simulink model "psd_db"  (R2020a)
settings: Solver=FixedStepDiscrete  StartTime=0.0  StopTime=inf  RelTol=1e-3
InitFcn:
  | spectrum_fft_setup;
  | load('data.mat');
libraries: simulink x3, hdlsllib x1
settings Model: DataTypeOverride=Off  Creator=rgb11127  LastModifiedBy=david
settings DataIOCC: SaveOutput=off  SaveTime=off  ReturnWorkspaceOutputs=off
settings OptimizationCC: BlockReduction=off  ConditionallyExecuteInputs=off  DefaultParameterBehavior=Inlined
settings DebuggingCC: AlgebraicLoopMsg=error  SingleTaskRateTransMsg=error  PregeneratedLibrarySubsystemCodeDiagnostic=none  ArithmeticOperatorsInVariantConditions=warning
settings HardwareCC: ProdBitPerPointer=32  ProdBitPerSizeT=32  ProdBitPerPtrDiffT=32  ProdLargestAtomicFloat=None  ProdIntDivRoundTo=Undefined  ProdEndianess=Unspecified  ProdWordSize=32  ProdHWDeviceType=ASIC/FPGA->ASIC/FPGA  TargetBitPerPointer=64  TargetBitPerSizeT=64  TargetBitPerPtrDiffT=64  TargetLongLongMode=on  TargetIntDivRoundTo=Zero  TargetEndianess=LittleEndian  TargetWordSize=64  TargetHWDeviceType=Custom Processor->MATLAB Host Computer  ProdEqTarget=off
settings SFSimCC: SimUseLocalCustomCode=off  CustomCodeUndefinedFunction=UseInterfaceOnly
settings RTWCC: RTWUseLocalCustomCode=off

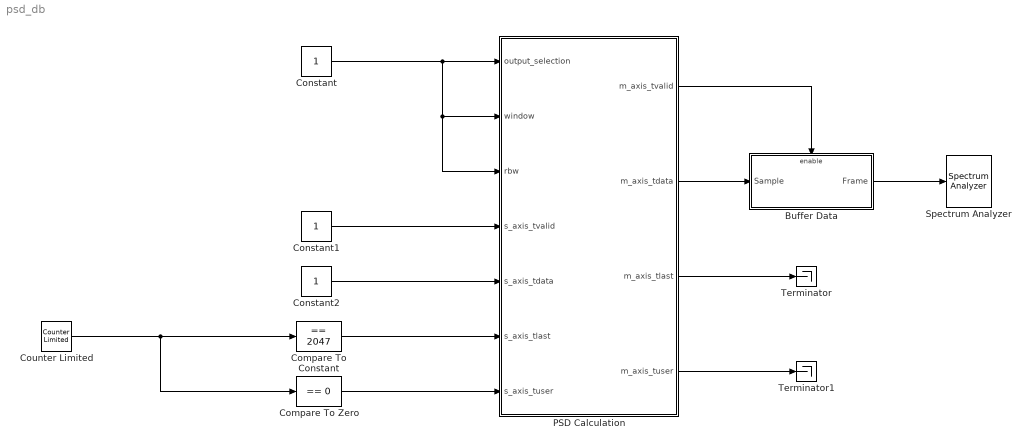
== system psd_db ==
  Buffer Data : Subsystem
  Compare To Constant : simulink/Logic and Bit Operations/Compare To Constant  relop===  const=2047  OutDataTypeStr=boolean
  Compare To Zero : simulink/Logic and Bit Operations/Compare To Zero  relop===  OutDataTypeStr=boolean
  Constant : Constant  OutDataTypeStr=uint32  SampleTime=1/256e6
  Constant1 : Constant  OutDataTypeStr=boolean  SampleTime=-1
  Constant2 : Constant  OutDataTypeStr=uint32  SampleTime=-1
  Counter Limited : simulink/Sources/Counter Limited  uplimit=2047  tsamp=-1
  PSD Calculation : Subsystem  TreatAsAtomicUnit=on
  Spectrum Analyzer : SpectrumAnalyzer  IsFrequencyInputMode=1
  Terminator : Terminator
  Terminator1 : Terminator
  wires:
  Constant/1 -> PSD Calculation/3(rbw), PSD Calculation/2(window), PSD Calculation/1(output_selection)
  PSD Calculation/2(m_axis_tdata) -> Buffer Data/1(Sample)
  PSD Calculation/1(m_axis_tvalid) -> Buffer Data/Enable
  PSD Calculation/3(m_axis_tlast) -> Terminator/1
  PSD Calculation/4(m_axis_tuser) -> Terminator1/1
  Counter Limited/1 -> Compare To Constant/1, Compare To Zero/1
  Compare To Constant/1 -> PSD Calculation/6(s_axis_tlast)
  Constant1/1 -> PSD Calculation/4(s_axis_tvalid)
  Buffer Data/1(Frame) -> Spectrum Analyzer/1
  Compare To Zero/1 -> PSD Calculation/7(s_axis_tuser)
  Constant2/1 -> PSD Calculation/5(s_axis_tdata)

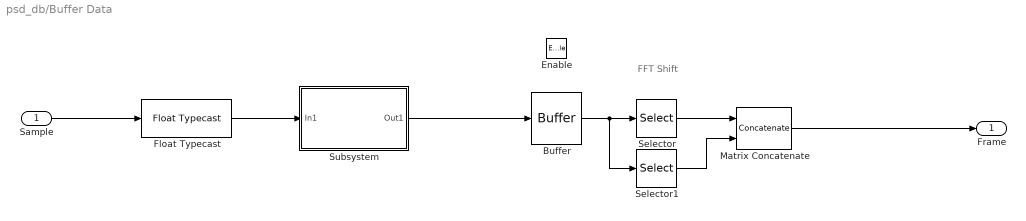
== system psd_db/Buffer Data ==
  note: FFT Shift
  Sample : Inport
  Enable : EnablePort
  Buffer : Buffer  N=2^11  OutputFrames=off
  Float Typecast : FloatTypecast
  Matrix Concatenate : Concatenate  Mode=Multidimensional array
  Selector : Selector  NumberOfDimensions=2  InputPortWidth=3  IndexOptions=Index vector (dialog),Index vector (dialog)  Indices=[1025:1:2048],1  OutputSizes=1,1
  Selector1 : Selector  NumberOfDimensions=2  InputPortWidth=3  IndexOptions=Index vector (dialog),Index vector (dialog)  Indices=[1:1:1024],1  OutputSizes=1,1
  Subsystem : Subsystem  Variant=on  VariantControlMode=Label  VariantControl=Variant1  LabelModeActiveChoice=Variant1
  Frame : Outport  VectorParamsAs1DForOutWhenUnconnected=off
  wires:
  Subsystem/1(" Out1") -> Buffer/1
  Sample/1 -> Float Typecast/1
  Selector1/1 -> Matrix Concatenate/2
  Matrix Concatenate/1 -> Frame/1
  Selector/1 -> Matrix Concatenate/1
  Buffer/1 -> Selector1/1, Selector/1
  Float Typecast/1 -> Subsystem/1("In1 ")

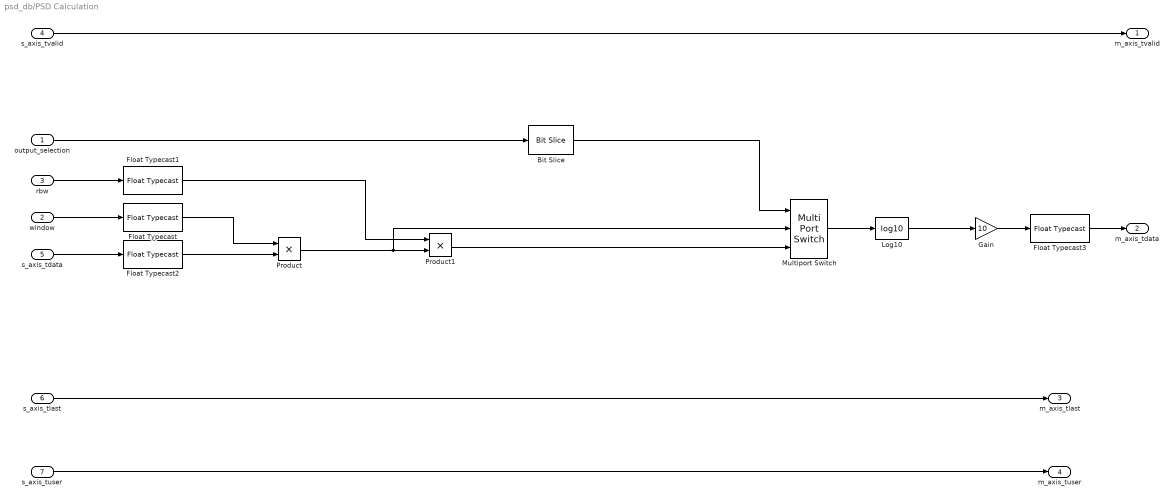
== system psd_db/PSD Calculation ==
  output_selection : Inport
  window : Inport  Port=2
  rbw : Inport  Port=3
  s_axis_tvalid : Inport  Port=4
  s_axis_tdata : Inport  Port=5
  s_axis_tlast : Inport  Port=6
  s_axis_tuser : Inport  Port=7
  Bit Slice : hdlsllib/Logic and Bit Operations/Bit Slice  lidx=0  ridx=0
      settings: SourceProductBaseCode=SL
  Float Typecast{,1..3} (4 alike) : FloatTypecast
  Gain : Gain  Gain=10
  Log10 : Math  Operator=log10  SignedPower=on  RndMeth=Zero  SaturateOnIntegerOverflow=on
  Multiport Switch : MultiPortSwitch  DataPortOrder=Zero-based contiguous  Inputs=2  zeroidx=on
  Product : Product
  Product1 : Product
  m_axis_tvalid : Outport  VectorParamsAs1DForOutWhenUnconnected=off
  m_axis_tdata : Outport  Port=2  VectorParamsAs1DForOutWhenUnconnected=off
  m_axis_tlast : Outport  Port=3  VectorParamsAs1DForOutWhenUnconnected=off
  m_axis_tuser : Outport  Port=4  VectorParamsAs1DForOutWhenUnconnected=off
  wires:
  Log10/1 -> Gain/1
  output_selection/1 -> Bit Slice/1
  s_axis_tvalid/1 -> m_axis_tvalid/1
  s_axis_tlast/1 -> m_axis_tlast/1
  s_axis_tuser/1 -> m_axis_tuser/1
  s_axis_tdata/1 -> Float Typecast2/1
  window/1 -> Float Typecast/1
  Float Typecast/1 -> Product/1
  Product/1 -> Multiport Switch/2, Product1/2
  Multiport Switch/1 -> Log10/1
  Gain/1 -> Float Typecast3/1
  Product1/1 -> Multiport Switch/3
  rbw/1 -> Float Typecast1/1
  Float Typecast1/1 -> Product1/1
  Bit Slice/1 -> Multiport Switch/1
  Float Typecast2/1 -> Product/2
  Float Typecast3/1 -> m_axis_tdata/1

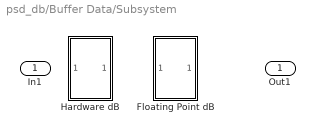
== system psd_db/Buffer Data/Subsystem ==
  "In1 " : Inport
  Floating Point dB : Subsystem  VariantControl=Variant
  Hardware dB : Subsystem  VariantControl=Variant1
  " Out1" : Outport  VectorParamsAs1DForOutWhenUnconnected=off

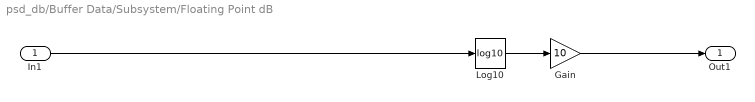
== system psd_db/Buffer Data/Subsystem/Floating Point dB ==
  In1 : Inport
  Gain : Gain  Gain=10
  Log10 : Math  Operator=log10  SignedPower=on  SaturateOnIntegerOverflow=on
  Out1 : Outport  VectorParamsAs1DForOutWhenUnconnected=off
  wires:
  In1/1 -> Log10/1
  Gain/1 -> Out1/1
  Log10/1 -> Gain/1

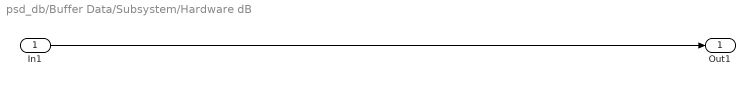
== system psd_db/Buffer Data/Subsystem/Hardware dB ==
  In1 : Inport
  Out1 : Outport  VectorParamsAs1DForOutWhenUnconnected=off
  wires:
  In1/1 -> Out1/1
